simulink model "mqr_example"  (R2019a)
settings: Solver=VariableStepAuto  StartTime=0.0  StopTime=100  RelTol=1e-3
undefined symbols (not defined in the file): den, num
settings Model: Creator=tarci  LastModifiedBy=PICHAU
settings DataIOCC: ReturnWorkspaceOutputs=off
settings DebuggingCC: ArithmeticOperatorsInVariantConditions=warning

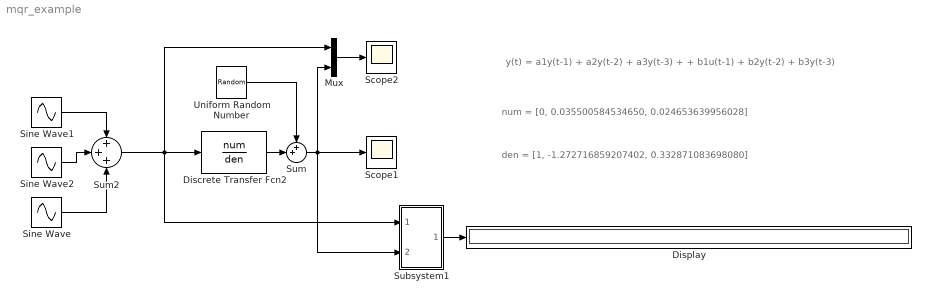
== system mqr_example ==
  note: y(t) = a1y(t-1) + a2y(t-2) + a3y(t-3) + + b1u(t-1) + b2y(t-2) + b3y(t-3)
  note: den = [1, -1.272716859207402, 0.332871083698080]
  note: num = [0, 0.035500584534650, 0.024653639956028]
  Discrete Transfer Fcn2 : DiscreteTransferFcn  Numerator=num  Denominator=den  SampleTime=0.1
  Display : Display
  Mux : Mux  Inputs=2
  Scope1 : Scope
  Scope2 : Scope
  Sine Wave : Sin  SampleTime=0
  Sine Wave1 : Sin  Amplitude=2  Frequency=0.5  SampleTime=0
  Sine Wave2 : Sin  Frequency=0.1  SampleTime=0
  Subsystem1 : Subsystem
  Sum : Sum  Inputs=++|
  Sum2 : Sum  Inputs=+++
  Uniform Random Number : UniformRandomNumber  Minimum=-0.01  Maximum=0.01  SampleTime=0.1
  wires:
  Subsystem1/1(Out1) -> Display/1
  Sum2/1 -> Mux/1, Subsystem1/1(In1), Discrete Transfer Fcn2/1
  Sum/1 -> Mux/2, Subsystem1/2(In2), Scope1/1
  Sine Wave1/1 -> Sum2/1
  Sine Wave2/1 -> Sum2/2
  Sine Wave/1 -> Sum2/3
  Uniform Random Number/1 -> Sum/1
  Discrete Transfer Fcn2/1 -> Sum/2
  Mux/1 -> Scope2/1

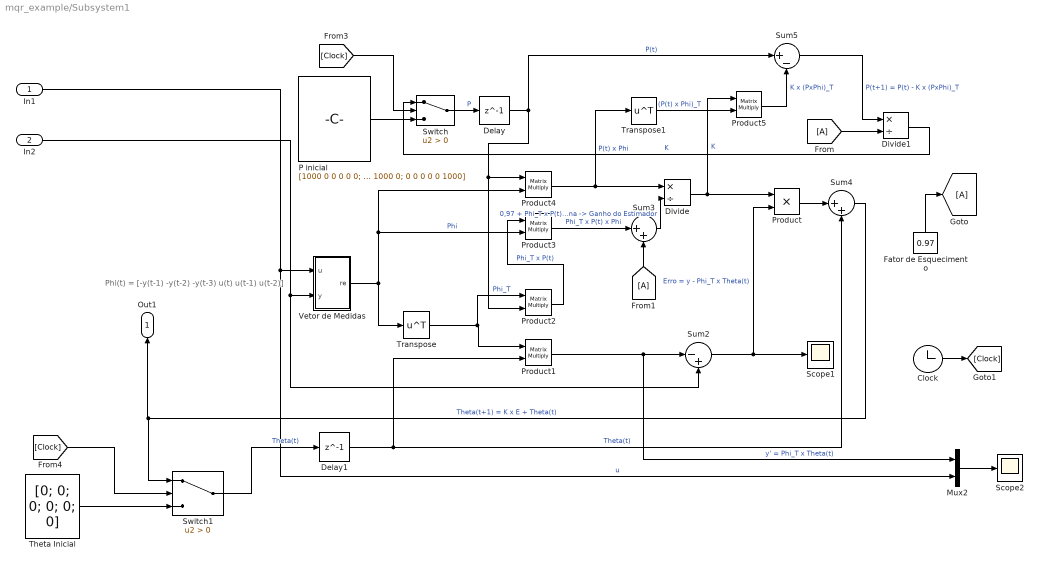
== system mqr_example/Subsystem1 ==
  note: Phi(t) = [-y(t-1) -y(t-2) -y(t-3) u(t) u(t-1) u(t-2)]
  In1 : Inport
  In2 : Inport  Port=2
  Clock : Clock
  Delay : Delay  DelayLength=1  InitialCondition=0  SampleTime=0.1
  Delay1 : Delay  DelayLength=1  InitialCondition=0  SampleTime=0.1
  Divide : Product  Inputs=*/
  Divide1 : Product  Inputs=*/
  "Fator de Esquecimento " : Constant  Value=0.97
  Mux2 : Mux  Inputs=2
  P inicial : Constant  Value=[1000 0 0 0 0 0; 0 1000 0 0 0 0; 0 0 1000 0 0 0; 0 0 0 1000 0 0; 0 0 0 0 1000 0; 0 0 0 0 0 1000]
  Product : Product
  Product{1..5} (5 alike) : Product  Multiplication=Matrix(*)
  Scope1 : Scope
  Scope2 : Scope
  Sum2 : Sum  Inputs=|-+
  Sum3 : Sum  Inputs=|++
  Sum4 : Sum  Inputs=|++
  Sum5 : Sum  Inputs=|+-
  Switch : Switch  Criteria=u2 > Threshold
  Switch1 : Switch  Criteria=u2 > Threshold
  "Theta Inicial " : Constant  Value=[0; 0; 0; 0; 0; 0]
  Transpose : Math  Operator=transpose  SaturateOnIntegerOverflow=on
  Transpose1 : Math  Operator=transpose  SaturateOnIntegerOverflow=on
  "Vetor de Medidas " : Subsystem
  Out1 : Outport
  wires:
  "Vetor de Medidas "/1(re) -> Transpose/1, Product4/2, Product3/2  "Phi"
  Product/1 -> Sum4/1
  In2/1 -> Sum2/2, "Vetor de Medidas "/2(y)
  "Fator de Esquecimento "/1 -> [A]
  Transpose/1 -> Product2/1, Product1/1  "Phi_T"
  Sum3/1 -> Divide/2  "0,97 + Phi_T x P(t) x Phi Vetor Coluna -> Ganho do Estimador"
  Product3/1 -> Sum3/1  "Phi_T x P(t) x Phi"
  Switch/1 -> Delay/1  "P"
  Product4/1 -> Transpose1/1, Divide/1  "P(t) x Phi"
  Delay/1 -> Product4/1, Product2/2, Sum5/1  "P(t)"
  Divide/1 -> Product5/1, Product/1  "K"
  Transpose1/1 -> Product5/2  "(P(t) x Phi)_T"
  Sum5/1 -> Divide1/1  "P(t+1) = P(t) - K x (PxPhi)_T"
  Sum2/1 -> Scope1/1, Product/2  "Erro = y - Phi_T x Theta(t)"
  Delay1/1 -> Sum4/2, Product1/2  "Theta(t)"
  Divide1/1 -> Switch/1  "K"
  "Theta Inicial "/1 -> Switch1/3
  [A] -> Divide1/2
  Product2/1 -> Product3/1  "Phi_T x P(t)"
  Clock/1 -> [Clock]
  Product1/1 -> Mux2/1, Sum2/1  "y' = Phi_T x Theta(t)"
  Product5/1 -> Sum5/2  "K x (PxPhi)_T"
  P inicial/1 -> Switch/3
  Sum4/1 -> Switch1/1, Out1/1  "Theta(t+1) = K x E + Theta(t)"
  [A] -> Sum3/2
  In1/1 -> Mux2/2, "Vetor de Medidas "/1(u)  "u"
  [Clock] -> Switch/2
  Switch1/1 -> Delay1/1  "Theta(t)"
  Mux2/1 -> Scope2/1
  [Clock] -> Switch1/2

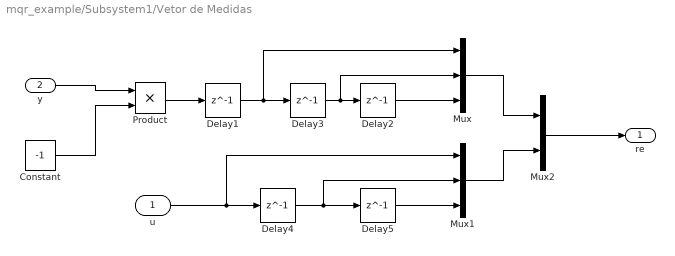
== system mqr_example/Subsystem1/Vetor de Medidas  ==
  u : Inport
  y : Inport  Port=2
  Constant : Constant  Value=-1
  Delay{1..5} (5 alike) : Delay  DelayLength=1  InitialCondition=0  SampleTime=0.1
  Mux : Mux  Inputs=3
  Mux1 : Mux  Inputs=3
  Mux2 : Mux  Inputs=2
  Product : Product
  re : Outport
  wires:
  Delay4/1 -> Mux1/2, Delay5/1
  Delay5/1 -> Mux1/3
  Mux1/1 -> Mux2/2
  Mux/1 -> Mux2/1
  Mux2/1 -> re/1
  u/1 -> Mux1/1, Delay4/1
  Delay2/1 -> Mux/3
  y/1 -> Product/1
  Constant/1 -> Product/2
  Product/1 -> Delay1/1
  Delay3/1 -> Mux/2, Delay2/1
  Delay1/1 -> Mux/1, Delay3/1
